simulink model "sim12ex1"  (Simulink 3.00)
settings: Solver=ode45  SolverMode=SingleTasking  StartTime=0.0  StopTime=10  MaxStep=.05  RelTol=1e-3  AbsTol=1e-3
settings Model: SaveTime=off  SaveOutput=off  RTWTemplateMakefile=grt_vc.tmf

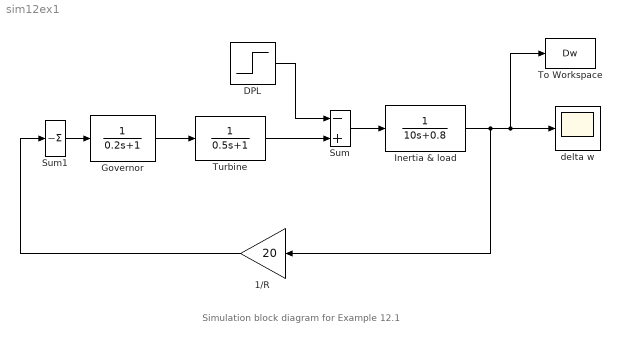
== system sim12ex1 ==
  note: Simulation block diagram for Example 12.1
  "   Governor" : TransferFcn  Numerator=[1]  Denominator="[0.2   1]"
  1/R : Gain  Orientation=left  Gain=20  SaturateOnIntegerOverflow=on
  "DPL " : Step  Time=0  Before=0  After=.2  SampleTime=0
  "Inertia & load " : TransferFcn  Numerator=[1]  Denominator="[10  0.8]"
  Sum : Sum  Inputs=-+  SaturateOnIntegerOverflow=on
  Sum1 : Sum  Inputs=-  SaturateOnIntegerOverflow=on
  To Workspace : ToWorkspace  VariableName=Dw  SampleTime=0  SaveFormat=Matrix
      settings: Buffer=1000
  Turbine : TransferFcn  Numerator=[1]  Denominator="[0.5  1]"
  delta w : Scope
      settings: TickLabels=on  TimeRange=10  YMin=-0.015  YMax=0  SaveToWorkspace=off  SaveName=ScopeData  DataFormat=Matrix
  wires:
  "DPL "/1 -> Sum/1
  "Inertia & load "/1 -> To Workspace/1, delta w/1, 1/R/1
  Sum1/1 -> "   Governor"/1
  Sum/1 -> "Inertia & load "/1
  Turbine/1 -> Sum/2
  "   Governor"/1 -> Turbine/1
  1/R/1 -> Sum1/1
